simulink model "CiMappedEngine"  (R2021b)
settings: Solver=VariableStepAuto  StartTime=0.0  StopTime=inf  RelTol=1e-3  EnableMultiTasking=on
model workspace (MAT data in the model file):
  AccPwrbp = Simulink.Parameter
  AccPwrbp.Value = [0 0]
  AccPwrbp.DataType = 'double'
  AccPwrbp.Complexity = 'real'
  AccPwrbp.Dimensions = [1 2]
  AccSpdbp = Simulink.Parameter
  AccSpdbp.Value = [300 750]
  AccSpdbp.DataType = 'double'
  AccSpdbp.Complexity = 'real'
  AccSpdbp.Dimensions = [1 2]
  Cps = Simulink.Parameter
  Cps.Value = 2
  Cps.DataType = 'double'
  Cps.Complexity = 'real'
  Cps.Dimensions = [1 1]
  NCyl = Simulink.Parameter
  NCyl.Value = 4
  NCyl.DataType = 'double'
  NCyl.Complexity = 'real'
  NCyl.Dimensions = [1 1]
  Pstd = Simulink.Parameter
  Pstd.Value = 101325
  Pstd.DataType = 'double'
  Pstd.Complexity = 'real'
  Pstd.Dimensions = [1 1]
  Rair = Simulink.Parameter
  Rair.Value = 287.05
  Rair.DataType = 'double'
  Rair.Complexity = 'real'
  Rair.Dimensions = [1 1]
  Sinj = Simulink.Parameter
  Sinj.Value = 6.45161290323
  Sinj.DataType = 'double'
  Sinj.Complexity = 'real'
  Sinj.Dimensions = [1 1]
  TimeCnstECP = Simulink.Parameter
  TimeCnstECP.Value = 0.125
  TimeCnstECP.DataType = 'double'
  TimeCnstECP.Complexity = 'real'
  TimeCnstECP.Dimensions = [1 1]
  TimeCnstEGR = Simulink.Parameter
  TimeCnstEGR.Value = 0.125
  TimeCnstEGR.DataType = 'double'
  TimeCnstEGR.Complexity = 'real'
  TimeCnstEGR.Dimensions = [1 1]
  TimeCnstETC = Simulink.Parameter
  TimeCnstETC.Value = 0.085
  TimeCnstETC.DataType = 'double'
  TimeCnstETC.Complexity = 'real'
  TimeCnstETC.Dimensions = [1 1]
  TimeCnstICP = Simulink.Parameter
  TimeCnstICP.Value = 0.125
  TimeCnstICP.DataType = 'double'
  TimeCnstICP.Complexity = 'real'
  TimeCnstICP.Dimensions = [1 1]
  TimeCnstIVL = Simulink.Parameter
  TimeCnstIVL.Value = 0.125
  TimeCnstIVL.DataType = 'double'
  TimeCnstIVL.Complexity = 'real'
  TimeCnstIVL.Dimensions = [1 1]
  TimeCnstSWVA = Simulink.Parameter
  TimeCnstSWVA.Value = 0.125
  TimeCnstSWVA.DataType = 'double'
  TimeCnstSWVA.Complexity = 'real'
  TimeCnstSWVA.Dimensions = [1 1]
  TimeCnstVCR = Simulink.Parameter
  TimeCnstVCR.Value = 0.125
  TimeCnstVCR.DataType = 'double'
  TimeCnstVCR.Complexity = 'real'
  TimeCnstVCR.Dimensions = [1 1]
  TimeCnstVGT = Simulink.Parameter
  TimeCnstVGT.Value = 0.15
  TimeCnstVGT.DataType = 'double'
  TimeCnstVGT.Complexity = 'real'
  TimeCnstVGT.Dimensions = [1 1]
  TimeCnstVIRL = Simulink.Parameter
  TimeCnstVIRL.Value = 0.125
  TimeCnstVIRL.DataType = 'double'
  TimeCnstVIRL.Complexity = 'real'
  TimeCnstVIRL.Dimensions = [1 1]
  TimeCnstWGA = Simulink.Parameter
  TimeCnstWGA.Value = 0.15
  TimeCnstWGA.DataType = 'double'
  TimeCnstWGA.Complexity = 'real'
  TimeCnstWGA.Dimensions = [1 1]
  Tstd = Simulink.Parameter
  Tstd.Value = 293.15
  Tstd.DataType = 'double'
  Tstd.Complexity = 'real'
  Tstd.Dimensions = [1 1]
  Vd = Simulink.Parameter
  Vd.Value = 0.0015
  Vd.DataType = 'double'
  Vd.Complexity = 'real'
  Vd.Dimensions = [1 1]
  f_air = Simulink.Parameter
  f_air.Value = [0 0 0 0 0 0 0 0 0 0 0 0 ... (320 elements, 20x16)]
  f_air.DataType = 'double'
  f_air.Complexity = 'real'
  f_air.Dimensions = [20 16]
  f_air_3d = Simulink.Parameter
  f_air_3d.Value = [0 0 0 0 0 0 0 0 0 0 0 0 ... (960 elements, 20x16x3)]
  f_air_3d.DataType = 'double'
  f_air_3d.Complexity = 'real'
  f_air_3d.Dimensions = [20 16 3]
  f_co = Simulink.Parameter
  f_co.Value = [0 0 0 0 0 0 0 0 0 0 0 0 ... (320 elements, 20x16)]
  f_co.DataType = 'double'
  f_co.Complexity = 'real'
  f_co.Dimensions = [20 16]
  f_co2 = Simulink.Parameter
  f_co2.Value = [0 0 0 0 0 0 0 0 0 0 0 0 ... (320 elements, 20x16)]
  f_co2.DataType = 'double'
  f_co2.Complexity = 'real'
  f_co2.Dimensions = [20 16]
  f_co2_3d = Simulink.Parameter
  f_co2_3d.Value = [0 0 0 0 0 0 0 0 0 0 0 0 ... (960 elements, 20x16x3)]
  f_co2_3d.DataType = 'double'
  f_co2_3d.Complexity = 'real'
  f_co2_3d.Dimensions = [20 16 3]
  f_co_3d = Simulink.Parameter
  f_co_3d.Value = [0 0 0 0 0 0 0 0 0 0 0 0 ... (960 elements, 20x16x3)]
  f_co_3d.DataType = 'double'
  f_co_3d.Complexity = 'real'
  f_co_3d.Dimensions = [20 16 3]
  f_eff = Simulink.Parameter
  f_eff.Value = [0 0 0 0 0 0 0 0 0 0 0 0 ... (320 elements, 20x16)]
  f_eff.DataType = 'double'
  f_eff.Complexity = 'real'
  f_eff.Dimensions = [20 16]
  f_eff_3d = Simulink.Parameter
  f_eff_3d.Value = [0 0 0 0 0 0 0 0 0 0 0 0 ... (960 elements, 20x16x3)]
  f_eff_3d.DataType = 'double'
  f_eff_3d.Complexity = 'real'
  f_eff_3d.Dimensions = [20 16 3]
  f_fuel = Simulink.Parameter
  f_fuel.Value = [0 0 0 0 0 0 0 0 0 0 0 0 ... (320 elements, 20x16)]
  f_fuel.DataType = 'double'
  f_fuel.Complexity = 'real'
  f_fuel.Dimensions = [20 16]
  f_fuel_3d = Simulink.Parameter
  f_fuel_3d.Value = [0 0 0 0 0 0 0 0 0 0 0 0 ... (960 elements, 20x16x3)]
  f_fuel_3d.DataType = 'double'
  f_fuel_3d.Complexity = 'real'
  f_fuel_3d.Dimensions = [20 16 3]
  f_hc = Simulink.Parameter
  f_hc.Value = [0 0 0 0 0 0 0 0 0 0 0 0 ... (320 elements, 20x16)]
  f_hc.DataType = 'double'
  f_hc.Complexity = 'real'
  f_hc.Dimensions = [20 16]
  f_hc_3d = Simulink.Parameter
  f_hc_3d.Value = [0 0 0 0 0 0 0 0 0 0 0 0 ... (960 elements, 20x16x3)]
  f_hc_3d.DataType = 'double'
  f_hc_3d.Complexity = 'real'
  f_hc_3d.Dimensions = [20 16 3]
  f_nox = Simulink.Parameter
  f_nox.Value = [0 0 0 0 0 0 0 0 0 0 0 0 ... (320 elements, 20x16)]
  f_nox.DataType = 'double'
  f_nox.Complexity = 'real'
  f_nox.Dimensions = [20 16]
  f_nox_3d = Simulink.Parameter
  f_nox_3d.Value = [0 0 0 0 0 0 0 0 0 0 0 0 ... (960 elements, 20x16x3)]
  f_nox_3d.DataType = 'double'
  f_nox_3d.Complexity = 'real'
  f_nox_3d.Dimensions = [20 16 3]
  f_pm = Simulink.Parameter
  f_pm.Value = [0  0  0  0  0  0  0  0  0  0  0  0  0  0  0  0; 0  0  0  0  0  0  0  0  0  0  0  0  0  0  0  0; 0  0  0  0  0  0  0  0  0  0  0  0  0  0  0  0; 0  0  0  0  0  0  0  0  0  0  0  0  0  0  0  0; 0  0  0  0  0  0  0  0  0  0  0  0  0  0  0  0; 0  0  0  0  0  0  0  0  0  0  0  0  0  0  0  0; 0  0  0  0  0  0  0  0  0  0  0  0  0  0  0  0; 0  0  0  0  0  0  0  0  0  0  0  0  0  0  0  0; 0  0  0  0  0  0  0  0  0  0  0  0  0  0  0  0; 0  0  0  0  0  0  0  0  0  0  0  0  0  0  0  0; 0  0  0  0  0  0  0  0  0  0  0  0  0  0  0  0; 0  0  0  0  0  0  0  0  0  0  0  0  0  0  0  0; 0  0  0  0  0  0  0  0  0  0  0  0  0  0  0  0; 0  0  0  0  0  0  0  0  0  0  0  0  0  0  0  0; 0  0  0  0  0  0  0  0  0  0  0  0  0  0  0  0; 0  0  0  0  0  0  0  0  0  0  0  0  0  0  0  0; 0  0  0  0  0  0  0  0  0  0  0  0  0  0  0  0; 0  0  0  0  0  0  0  0  0  0  0  0  0  0  0  0; 0  0  0  0  0  0  0  0  0  0  0  0  0  0  0  0; 0  0  0  0  0  0  0  0  0  0  0  0  0  0  0  0]
  f_pm.DataType = 'double'
  f_pm.Complexity = 'real'
  f_pm.Dimensions = [20 16]
  f_pm_3d = Simulink.Parameter
  f_pm_3d.Value = reshape([0 0 0 0 0 0 0 0 0 0 0 0 0 0 0 0 0 0 0 0 0 0 0 0 0 0 0 0 0 0 0 0 0 0 0 0 0 0 0 0 0 0 0 0 0 0 0 0 0 0 0 0 0 0 0 0 0 0 0 0 0 0 0 0 0 0 0 0 0 0 0 0 0 0 0 0 0 0 0 0 0 0 0 0 0 0 0 0 0 0 0 0 0 0 0 0 0 0 0 0 0 0 0 0 0 0 0 0 0 0 0 0 0 0 0 0 0 0 0 0 0 0 0 0 0 0 0 0 0 0 0 0 0 0 0 0 0 0 0 0 0 0 0 0 0 0 0 0 0 0 0 0 0 0 0 0 0 0 0 0 0 0 0 0 0 0 0 0 0 0 0 0 0 0 0 0 0 0 0 0 0 0 0 0 0 0 0 0 0 0 0 0 0 0 0 0 0 0 0 0 0 0 0 0 0 0 0 0 0 0 0 0 0 0 0 0 0 0 0 0 0 0 0 0 0 0 0 0 0 0 0 0 0 0 0 0 0 0 0 0 0 0 0 0 0 0 0 0 0 0 0 0 0 0 0 0 0 0 0 0 0 0 0 0 0 0 0 0 0 0 0 0 0 0 0 0 0 0 0 0 0 0 0 0 0 0 0 0 0 0 0 0 0 0 0 0 0 0 0 0 0 0 0 0 0 0 0 0 0 0 0 0 0 0 0 0 0 0 0 0 0 0 0 0 0 0 0 0 0 0 0 0 0 0 0 0 0 0 0 0 0 0 0 0 0 0 0 0 0 0 0 0 0 0 0 0 0 0 0 0 0 0 0 0 0 0 0 0 0 0 0 0 0 0 0 0 0 0 0 0 0 0 0 0 0 0 0 0 0 0 0 0 0 0 0 0 0 0 0 0 0 0 0 0 0 0 0 0 0 0 0 0 0 0 0 0 0 0 0 0 0 0 0 0 0 0 0 0 0 0 0 0 0 0 0 0 0 0 0 0 0 0 0 0 0 0 0 0 0 0 0 0 0 0 0 0 0 0 0 0 0 0 0 0 0 0 0 0 0 0 0 0 0 0 0 0 0 0 0 0 0 0 0 0 0 0 0 0 0 0 0 0 0 0 0 0 0 0 0 0 0 0 0 0 0 0 0 0 0 0 0 0 0 0 0 0 0 0 0 0 0 0 0 0 0 0 0 0 0 0 0 0 0 0 0 0 0 0 0 0 0 0 0 0 0 0 0 0 0 0 0 0 0 0 0 0 0 0 0 0 0 0 0 0 0 0 0 0 0 0 0 0 0 0 0 0 0 0 0 0 0 0 0 0 0 0 0 0 0 0 0 0 0 0 0 0 0 0 0 0 0 0 0 0 0 0 0 0 0 0 0 0 0 0 0 0 0 0 0 0 0 0 0 0 0 0 0 0 0 0 0 0 0 0 0 0 0 0 0 0 0 0 0 0 0 0 0 0 0 0 0 0 0 0 0 0 0 0 0 0 0 0 0 0 0 0 0 0 0 0 0 0 0 0 0 0 0 0 0 0 0 0 0 0 0 0 0 0 0 0 0 0 0 0 0 0 0 0 0 0 0 0 0 0 0 0 0 0 0 0 0 0 0 0 0 0 0 0 0 0 0 0 0 0 0 0 0 0 0 0 0 0 0 0 0 0 0 0 0 0 0 0 0 0 0 0 0 0 0 0 0 0 0 0 0 0 0 0 0 0 0 0 0 0 0 0 0 0 0 0 0 0 0 0 0 0 0 0 0 0 0 0 0 0 0 0 0 0 0 0 0 0 0 0 0 0 0 0 0 0 0 0 0 0 0 0 0 0 0 0 0 0 0 0 0 0 0 0 0 0 0 0 0 0 0 0 0 0 0 0 0 0 0 0 0 0 0 0 0 0 0 0 0 0 0 0 0 0 0 0 0 0 0 0 0 0 0 0 0 0 0 0 0 0 0 0 0 0 0 0 0 0 0 0 0 0 0 0 0 0 0 0 0 0 0 0 0 0 0 0 0 0 0 0 0 0 0 0 0 0 0 0 0 0 0 0 0 0 0 0 0 0 0 0 0 0 0 0 0 0 0 0 0 0 0 0 0 0 0 0 0 0 0 0 0 0 0 0 0 0 0 0 0 0 0 0 0 0 0 0 0 0 0 0 0 0 0 0 0 0], [20 16 3])
  f_pm_3d.DataType = 'double'
  f_pm_3d.Complexity = 'real'
  f_pm_3d.Dimensions = [20 16 3]
  f_tbrake = Simulink.Parameter
  f_tbrake.Value = [0 15 15 15 15 15 15 15 15 15 15 15 ... (320 elements, 20x16)]
  f_tbrake.DataType = 'double'
  f_tbrake.Complexity = 'real'
  f_tbrake.Dimensions = [20 16]
  f_tbrake_3d = Simulink.Parameter
  f_tbrake_3d.Value = [0 4.32139921766 20.7572447114 35.9627269415 49.855265726 62.5657141177 74.4770044016 86.1003984024 97.7334079818 109.479762957 121.326441846 133.101497884 ... (960 elements, 20x16x3)]
  f_tbrake_3d.DataType = 'double'
  f_tbrake_3d.Complexity = 'real'
  f_tbrake_3d.Dimensions = [20 16 3]
  f_tbrake_f_bpt = Simulink.Parameter
  f_tbrake_f_bpt.Value = [0 2.63157894737 5.26315789474 7.89473684211 10.5263157895 13.1578947368 15.7894736842 18.4210526316 21.0526315789 23.6842105263 26.3157894737 28.9473684211 31.5789473684 34.2105263158 36.8421052632 39.4736842105 42.1052631579 44.7368421053 47.3684210526 50]
  f_tbrake_f_bpt.DataType = 'double'
  f_tbrake_f_bpt.Complexity = 'real'
  f_tbrake_f_bpt.Dimensions = [1 20]
  f_tbrake_n_bpt = Simulink.Parameter
  f_tbrake_n_bpt.Value = [0 1000 1285.71428571 1571.42857143 1857.14285714 2142.85714286 2428.57142857 2714.28571429 3000 3285.71428571 3571.42857143 3857.14285714 4142.85714286 4428.57142857 4714.28571429 5000]
  f_tbrake_n_bpt.DataType = 'double'
  f_tbrake_n_bpt.Complexity = 'real'
  f_tbrake_n_bpt.Dimensions = [1 16]
  f_tbrake_t_bpt = Simulink.Parameter
  f_tbrake_t_bpt.Value = [0 4.017 21.26 37.37 52.22 65.88 78.77 91.44 104.2 116.8 129.3 141.4 153.4 165.7 178.4 191.7 205.6 219.7 233.5 246.7]
  f_tbrake_t_bpt.DataType = 'double'
  f_tbrake_t_bpt.Complexity = 'real'
  f_tbrake_t_bpt.Dimensions = [1 20]
  f_texh = Simulink.Parameter
  f_texh.Value = [530.615953519 585.141308787 621.791548793 637.74644696 668.027558986 729.99378178 762.870339995 814.420601609 844.420048857 859.04703204 894.926983859 943.665474082 ... (320 elements, 20x16)]
  f_texh.DataType = 'double'
  f_texh.Complexity = 'real'
  f_texh.Dimensions = [20 16]
  f_texh_3d = Simulink.Parameter
  f_texh_3d.Value = [358.711368346 410.521929896 465.556483184 518.480956339 566.158596806 618.256764358 675.886138918 720.044246232 742.940029896 751.128194054 760.390444558 779.777710435 ... (960 elements, 20x16x3)]
  f_texh_3d.DataType = 'double'
  f_texh_3d.Complexity = 'real'
  f_texh_3d.Dimensions = [20 16 3]
libraries: autolibpowerinfoutils x1, autolibsharedmappedengines x1
(part 1 of 2)
settings Model: DataDictionary=CiMappedEngine.sldd  ModifiedByFormat=The MathWorks, Inc.  Creator=The MathWorks, Inc.  LastModifiedBy=The MathWorks, Inc.
settings SolverCC: AlgebraicLoopSolver=TrustRegion  DecoupledContinuousIntegration=on
settings DataIOCC: DSMLogging=off  ReturnWorkspaceOutputs=off
settings DebuggingCC: SFMachineParentedDataDiag=warning  ArithmeticOperatorsInVariantConditions=warning
settings SFSimCC: SimUseLocalCustomCode=off  CustomCodeUndefinedFunction=UseInterfaceOnly
settings RTWCC: RTWUseLocalCustomCode=off
settings CodeAppCC: StateflowObjectComments=on
settings GRTTargetCC: TargetLangStandard=C89/C90 (ANSI)
settings ConfigComp: CovMetricSettings=dsw  CovSaveCumulativeToWorkspaceVar=on  CovSaveSingleToWorkspaceVar=on  CovExternalEMLEnable=off
settings SimscapeCC: SimscapeNormalizeSystem=off  SimscapeNominalValues={1, 'bar'; 1, 'cm^3/s'; 1, 'bar*kg/s'; 1, 'kJ/kg'; 1, 'kW'}

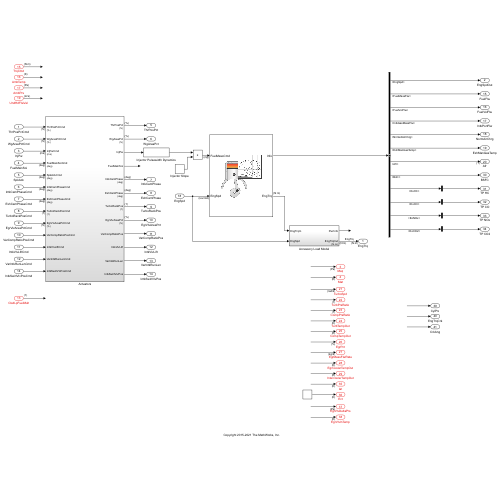
[thumbnail: Simulink's stored preview of the top-level diagram]
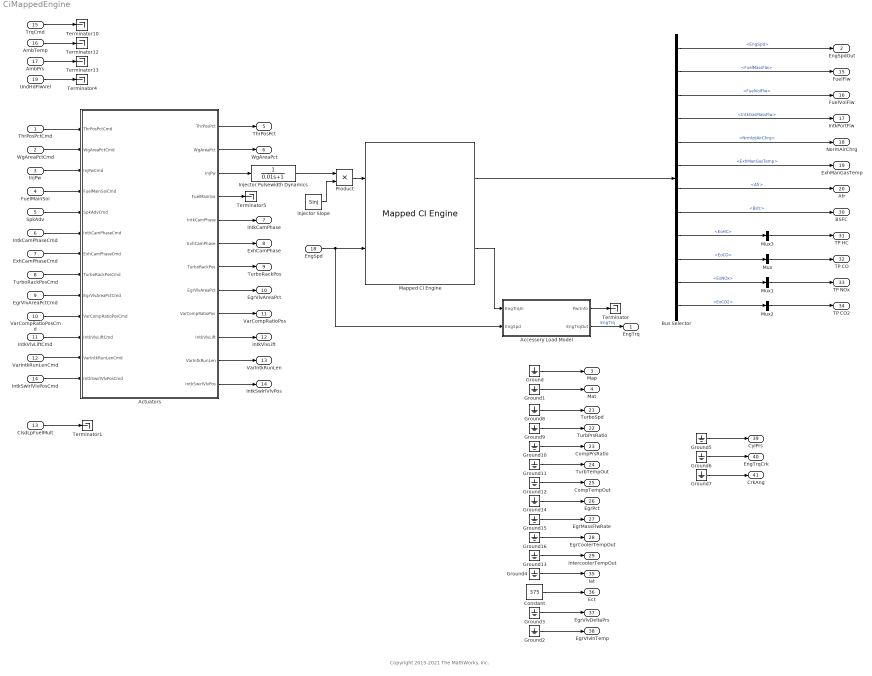
== system CiMappedEngine ==
  note: Copyright 2015-2021 The MathWorks, Inc.
  ThrPosPctCmd : Inport
  WgAreaPctCmd : Inport  Port=2
  InjPw : Inport  Port=3
  FuelMainSoi : Inport  Port=4
  SpkAdv : Inport  Port=5
  IntkCamPhaseCmd : Inport  Port=6
  ExhCamPhaseCmd : Inport  Port=7
  TurboRackPosCmd : Inport  Port=8
  EgrVlvAreaPctCmd : Inport  Port=9
  VarCompRatioPosCmd : Inport  Port=10
  IntkVlvLiftCmd : Inport  Port=11
  VarIntkRunLenCmd : Inport  Port=12
  ClsdLpFuelMult : Inport  Port=13  Unit=1
  IntkSwirlVlvPosCmd : Inport  Port=14
  TrqCmd : Inport  Port=15  Unit=N*m
  AmbTemp : Inport  Port=16  Unit=K
  AmbPrs : Inport  Port=17  Unit=Pa
  EngSpd : Inport  Port=18  Interpolate=off
  UndHdFlwVel : Inport  Port=19  Unit=m/s
  Accessory Load Model : Subsystem
  Actuators : Subsystem
  Bus Selector : BusSelector  OutputSignals=EngSpd,FuelMassFlw,FuelVolFlw,IntkGasMassFlw,NrmlzdAirChrg,ExhManGasTemp,Afr,Bsfc,EoHC,EoCO,EoNOx,EoCO2
  Constant : Constant  Value=375
  Ground{,1..16} (17 alike) : Ground
  Injector Pulsewidth Dynamics : TransferFcn  Denominator=[0.01 1]
  Injector Slope : Constant  Value=Sinj
  Mapped CI Engine : autolibsharedmappedengines/Mapped CI Engine  InputCmdPopup=Fuel mass  TurboLagCheckbox=off  EngTmpInpEnbl=off  rowVarName=TrqCmd  f_tbrake_f_bpt=f_tbrake_f_bpt  f_tbrake_t_bpt=f_tbrake_t_bpt  colVarName=EngSpd  f_tbrake_n_bpt=f_tbrake_n_bpt  f_tbrake_engtmp_bpt=[0 1000 1285.71428571429 1571.42857142857 1857.14285714286 2142.85714285714 2428.57142857143 2714.28571428571 3000 3285.71428571429 3571.42857142857 3857.14285714286 4142.85714285714 4428.57142857143 4714.28571428571 5000]  NCyl=NCyl  Cps=Cps  Vd=Vd  Lhv=45e6  Sg=0.832  Rair=Rair  Pstd=Pstd  Tstd=Tstd  Use1=on  Use2=on  Use3=on  Use4=on  Use5=on  Use6=on  Use7=on  Use8=on  Use9=on  Use10=off  f_tbrake_bst=[90, 95, 95, 95, 96, 100, 104, 104, 104, 100, 95, 85, 75, 67, 60, 55]  tau_nat=0.1  tau_bst_rising=1.0  tau_bst_falling=0.7  f_blend_frac=0.01  Name1=Brake Torque  f_tbrake=f_tbrake  f_tbrake_3d=cat(3,[0 -13.1081458684774 -14.1037949635308 -15.5978222223895 -17.1468243988479 -18.57688227287 -19.9284644067992 -21.2542794863055 -22.5937120686825 -24.0017516696912 -25.5203729932636 -27.1667334739623 -28.9776139270543 -31.0652059053262 -33.6382508909905 -36.9873078874202;4.32139921766168 4.32139921766168 4.01696946242645 3.01657627710533 1.85358637804622 0.731516929734549 -0.4275387192502 -1.6561494194378 -2.95770994431816 -4.36637302182332 -5.88102944693574 -7.45086843033805 -9.05557392067087 -10.7763270640777 -12.796196773429 -15.3493054793365;20.757244711379 20.757244711379 21.2571513067777 20.7978892952266 19.9910981679013 19.1178286650763 18.1132099278104 16.9543909701551 15.6490277189844 14.1813864135569 12.6063311068736 11.047099076305 9.56356301296286 8.06856710184566 6.37897429143581 4.32789906798446;35.9627269414642 35.9627269414642 37.3688456485072 37.4967194297404 37.0204872778024 36.3613948045835 35.5253088841127 34.4682997931625 33.1775441596392 31.6622717238732 30.0361023542073 28.4879672009938 27.0975462675126 25.7330173462773 24.1825303780978 22.3468615101609;49.8552657259726 49.8552657259726 52.2167310328196 52.9733200758864 52.8662249930047 52.4835369255407 51.8917326649162 51.0033454025654 49.7832430749781 48.2789577545489 46.6575307752233 45.1520123081703 43.8459468590103 42.5572123684317 41.0363966513775 39.2223005091444;62.5657141177372 62.5657141177372 65.8831947231727 67.3435083597075 67.7482462698726 67.8043747818398 67.5850553575219 66.9435552010083 65.8425982505031 64.3910827013451 62.8078461464009 61.3518293888112 60.1077185922706 58.8589256293869 57.319516534669 55.4366133009561;74.477004401576 74.477004401576 78.7701323679482 81.0576508161983 82.1550115553721 82.8010970398817 83.0434289470775 82.6817940293035 81.6963304630852 80.2758690996741 78.6966647443712 77.2463474522679 76.0244210658268 74.7962055302467 73.2304818257695 71.2491878151604;86.1003984024147 86.1003984024147 91.4403848598737 94.6662578802864 96.5423763308834 97.7951601239239 98.4662457785871 98.3255389688887 97.3704373723042 95.8764879743608 94.2178248871414 92.7449049403045 91.560940932338 90.3786230785299 88.8022437200717 86.7312355288638;97.7334079817966 97.7334079817966 104.159640567149 108.333038149937 110.951645304697 112.751774515793 113.767119577956 113.736058315812 112.652011363998 110.885495354204 109.00563172831 107.50897096566 106.468900898909 105.447451722756 103.936744797267 101.836124688201;109.479762957418 109.479762957418 116.819239580331 121.785496063185 125.100419113855 127.517149489911 128.937109713723 128.978763347179 127.598490805448 125.286894087135 122.924794214455 121.283173749861 120.428652893331 119.688104302635 118.358109739931 116.328046918923;121.326441846396 121.326441846396 129.256746784122 134.801128987357 138.834183316905 142.084246404129 144.125534715133 144.323033261273 142.583968288345 139.561104144292 136.474675856478 134.450177681175 133.638504705164 133.121882385945 131.951673587603 130.013338129768;133.101497884419 133.101497884419 141.390423214992 147.492975799703 152.341446310031 156.513845250296 159.270404298858 159.701130755565 157.676228517122 154.055833011852 150.345084498928 147.936876100182 147.055031208233 146.57504282138 145.352051741223 143.327096283665;144.820899208063 144.820899208063 153.421621226276 160.170390947986 165.811081311634 170.679187177046 174.011429217703 174.723297653528 172.66129491056 168.876865408438 165.011029375467 162.478515988541 161.481832233675 160.830603115659 159.333139273686 157.000941329443;156.736480114968 156.736480114968 165.665608236336 172.981857305465 179.187187414613 184.464635460139 188.162745737646 189.162853683952 187.38585429464 184.016652748413 180.526272843455 178.002164899037 176.608934842436 175.45436155568 173.584473896243 170.951232344112;169.114710642361 169.114710642361 178.391434699741 186.176266646156 192.786027371817 198.285653474534 202.073246296265 203.186779695165 201.750788334907 198.96643821215 195.929170221711 ...(+12274 chars)])  Name2=Air Mass Flow  f_air=f_air  f_air_3d=cat(3,[0 0.00309706924950592 0.00452015548895638 0.00626693492213078 0.00879912183278348 0.0118780141352622 0.0146086872326241 0.0164283363560914 0.017430833463342 0.0179780359688698 0.0183296451622608 0.0185647242912905 0.0186520238218037 0.0185206414129648 0.0181086367688216 0.0174012027671944;0 0.00602292528585861 0.00770048695740641 0.00909327842187188 0.0120300250825315 0.0165547686351833 0.0195929621698111 0.0205166972641812 0.0205599898366506 0.0207203034276991 0.0211816497894974 0.0218000682616549 0.0224177900393616 0.0228313059997907 0.022838545013414 0.0223621006077339;0 0.00872840998619654 0.0119344185519278 0.0150347158665953 0.0186401194316719 0.0220516764842476 0.0232455963198542 0.0227496747610248 0.022315206695101 0.0227059865534211 0.0235552063657731 0.0247029468037314 0.0262251280736842 0.0276235809443034 0.0283154367096376 0.0283212514239343;0 0.0104882072017092 0.0149369369892934 0.0194071452576307 0.0234570953719028 0.0264743743207795 0.0278624533425652 0.0279142745177744 0.0275369343940129 0.0274156787405589 0.0276419826170279 0.028751250915015 0.0310753059304267 0.0334431313520856 0.0347160350646922 0.0352041887413915;0 0.011712168284924 0.0163701147244402 0.0205936040826631 0.024568631705785 0.0286183696627147 0.0321435952324048 0.034217055691985 0.0347312239715439 0.034496131683675 0.0346154869246281 0.0357155943731093 0.0376532165828575 0.0397890303933338 0.041465041333155 0.0422265141888633;0 0.0118312143050573 0.0161536266038965 0.0199257826871529 0.0236447392965077 0.0278874214850712 0.0320911410431683 0.0355319414463786 0.0381473109012507 0.0402474553755304 0.0418777340103424 0.0430635720676062 0.044104298120767 0.0452740851072815 0.0464766914282441 0.0473016169107081;0 0.0110465687603505 0.0147448001879976 0.0186982152653005 0.0233180272070577 0.02848967544271 0.0332213005321568 0.0370211588830352 0.0405545130029438 0.044572205134237 0.0483929460850711 0.0506432109795243 0.0511287512595987 0.0512056237163403 0.0520782826150034 0.0532844037021472;0 0.0104431005689455 0.0140412319781156 0.0186656040327574 0.0243808115038222 0.0304790901592309 0.0358563735218778 0.0398156150298808 0.0431173259508535 0.0469471574428406 0.0509987494297762 0.0536398238059855 0.0543064471273892 0.0546047048338575 0.056061016585052 0.0580171322968633;0 0.0108025838625983 0.0147329075783379 0.0199272160885801 0.0269494950175881 0.0350856622579705 0.0423805976180197 0.0475930434283361 0.0511546617444798 0.0538624225439131 0.0553835460317609 0.0555838102527836 0.0555667873119217 0.056594819532664 0.0588984420072796 0.0617150043278395;0 0.01183615404291 0.015579473332316 0.0207476894033608 0.0291566563357895 0.0404435443970542 0.0507984356999528 0.0587530704305265 0.0649619731202889 0.0698463364144272 0.0724789010286908 0.0725501004086276 0.0711596039900798 0.0695425955723599 0.0686753046594181 0.0693454311429488;0 0.0127240149300819 0.0166943434305672 0.0213167267720966 0.0289502837647639 0.0400653409995224 0.0513974226551378 0.0604623088982535 0.0678845803192903 0.0753268542302593 0.0820105776211095 0.0855945811173189 0.0853773765956796 0.0831281579249428 0.081073849758615 0.080081315740193;0 0.0110641453709759 0.0153408643765708 0.0205300836592455 0.0288449359807962 0.0405948104237211 0.0521701453289181 0.0615930540891253 0.0695902332854493 0.0773195773497623 0.0841151408595659 0.088334695168896 0.089836067046592 0.0903700280065862 0.0909243501674699 0.0904976630313823;0 0.00833019140075226 0.0135692203293849 0.0205158026876127 0.029849570119091 0.040810538170541 0.0510111942628966 0.0598705369646537 0.0681187978770399 0.0760999983843794 0.0825339047146241 0.0867122889636778 0.0895837553206919 0.0920372076390418 0.0940819738186311 0.0954699432157815;0 0.00655239324915465 0.0124582375744647 0.019731165806625 0.0283852357889038 0.038223674378621 0.049417712197541 0.0598093990036953 0.0683274458944638 0.075112746920361 0.0800000023035051 0.0829602155432646 0.0850309276879992 0.0876816601880811 0.0912763887167288 ...(+13141 chars)])  Name3=Fuel Flow  f_fuel=f_fuel  f_fuel_3d=cat(3,[0 0 0 0 0 0 1.96872590895162e-08 1.11497559089192e-07 2.08845127798106e-07 2.82196894845497e-07 3.36789183807035e-07 3.85963069087249e-07 4.43703799512474e-07 5.16303552365966e-07 6.18958920559444e-07 7.66022406381668e-07;0 8.65785362426501e-05 0.00011203764940267 0.000137411179243721 0.00016270746005005 0.000187945932561446 0.00021312794139946 0.0002382669520308 0.000263366151267778 0.000288441610892002 0.000313504671335018 0.000338563835699193 0.000363629535167578 0.000388708193714062 0.000413810734167462 0.000438953321603612;0 0.000174726035507858 0.000225152899075032 0.000275508155686899 0.000325799742757026 0.000376033006192685 0.000426224614562359 0.000476378444759466 0.00052650775641107 0.00057661136482858 0.000626701339027024 0.000676788018376088 0.000726877918663027 0.000776982406974879 0.000827105108458734 0.000877258289084099;0 0.000262751467992024 0.00033815711141714 0.000413509147749243 0.000488810553518419 0.000564063749931979 0.00063928056610551 0.000714470811260552 0.000789634562401864 0.000864779715478911 0.00093991739471757 0.00101505165767627 0.00109018850480272 0.00116533546923552 0.00124049316997444 0.00131567174054954;0 0.000350674622437212 0.000451079528986024 0.000551436546045139 0.000651750832933373 0.000752042172469353 0.000852303056689121 0.00095253536480496 0.00105275214616171 0.00115295860006142 0.0012531576082591 0.00135334897972371 0.00145354034681151 0.00155374157057415 0.00165395024017036 0.00175417640620197;0 0.000438523155398598 0.000563925299253614 0.00068929628290271 0.000814645829677503 0.000939976999036283 0.001065288419702 0.00119058587147412 0.0013158694017402 0.00144114084528669 0.00156640851566576 0.0016916722751574 0.00181693265390974 0.00194219580045656 0.00206746569238982 0.00219275425952363;0 0.000526315425106774 0.000676728986990437 0.000827125576794928 0.000977509956968386 0.00112788874103488 0.00127826025858348 0.00142862216689251 0.00157897837839604 0.00172932766397965 0.00187967288170457 0.00203001238929626 0.00218034633484077 0.00233068458827493 0.00248102887035893 0.00263137738480869;0 0.000614090293790132 0.000789508746068303 0.000964932673154394 0.00114036147974239 0.00131579049815924 0.00149122146693545 0.00166665161834229 0.0018420830255848 0.00201751320081695 0.00219293915270003 0.00236836178159738 0.00254378375898177 0.00271920464503755 0.00289462481590337 0.00307005046750055;0 0.000701854437168888 0.000902286333293199 0.00110273789235218 0.00130320355815633 0.00150368554903504 0.00170418578418384 0.00190468941205035 0.00210519697462961 0.00230570553537478 0.0025062157636349 0.00270672441780583 0.00290722747290807 0.00310772903092585 0.00330823075338495 0.00350873484232527;0 0.000789649340075805 0.0010150845509588 0.00124055848345417 0.00146606558137245 0.00169159899277097 0.00191715641046872 0.00214272626450072 0.00236830926864185 0.00259390116245577 0.00281949040707559 0.00304508145248784 0.00327067513685969 0.00349626254985207 0.00372184957344385 0.0039474323233373;0 0.000877488592369892 0.00112793274528237 0.00137842091388439 0.00162895825749475 0.00187953790343879 0.00213014403908549 0.0023807781378913 0.00263143096817038 0.00288209397350937 0.0031327661795019 0.00338344231576459 0.00363411526528075 0.00388478536124402 0.00413545265696539 0.00438611177099695;0 0.000965411294698122 0.00124084233073851 0.00151633453527839 0.0017918942582486 0.00206750600688409 0.00234316285075658 0.00261885261867168 0.00289456620925925 0.00317029654400497 0.00344604094255091 0.00372179266401898 0.00399754312534031 0.00427329087379054 0.00454903339486812 0.00482476409430018;0 0.0010534117250146 0.00135382536745709 0.00165432071941838 0.00195489381219168 0.0022555293855071 0.00255621411457967 0.00285694714347189 0.00315771657791031 0.00345850732940484 0.00375931514196172 0.00406013514206826 0.00436095638616358 0.0046617732232831 0.00496258457239849 0.00526338302180174;0 0.00114152016247886 0.00146691663641427 0.00179239333752689 0.00211796534690249 0.00244360868792483 ...(+13971 chars)])  Name4=Exhaust Temperature  f_texh=f_texh  f_texh_3d=cat(3,[358.711368346279 358.711368346279 367.983969839492 375.766236578521 379.824873013623 380.377581918888 381.168020674094 384.445628826361 389.975238414473 397.276334747317 406.687273458426 418.723655106797 433.343123892387 449.95713948592 467.887943023565 486.766068837338;410.521929895625 410.521929895625 418.333326741241 425.972726120476 430.142630320378 430.676036782825 433.565609920626 439.830692307499 446.677697654088 452.935492545412 459.921840004908 469.184147095924 481.106853505583 495.16688690855 510.625205052308 527.104289154894;465.556483183975 465.556483183975 470.789185946812 475.838502443986 480.295227783728 485.406910889802 495.495051944124 508.573634165955 519.57749983902 526.850757499387 532.455117721457 538.704931547602 546.67711884581 556.710936307477 568.417449771026 581.104011694485;518.480956338607 518.480956338607 520.899294741741 523.582135138291 528.595311716542 536.846832033099 550.734399138879 568.993556445828 586.848331191129 600.477075260956 609.4895047716 615.505834518885 620.86855927714 627.910927144035 637.072100901679 647.109616946413;566.158596806175 566.158596806175 567.687323012922 572.746317112909 580.726768000975 588.013457446177 597.926992283215 614.220587792806 634.624060621759 653.584855786604 667.720901691748 677.333709356163 684.916260551597 693.10564253556 702.779084224323 713.371213106786;618.256764358386 618.256764358386 624.477092679185 633.413924976204 641.337589870685 643.8930379857 648.163836293112 659.880379116932 675.9331795421 690.676983743342 703.48679807145 716.671213932218 730.807374933275 744.672663864793 757.311023892644 769.273185572513;675.886138917862 675.886138917862 690.728265001459 698.761147883829 697.795213788686 691.167357063837 691.393891761148 702.947342129308 717.508872010719 726.807220251821 733.985585412432 746.79008634134 766.115681043826 785.866956815865 801.125878987934 813.153434705284;720.044246232086 720.044246232086 742.866930253765 747.250964575908 735.027333656649 719.577465323261 717.190065288522 731.346650709908 750.347138521549 763.475345837109 773.693695717131 789.287798577171 810.518185319644 830.111125982765 843.472450346469 853.378699854974;742.940029895664 742.940029895664 774.051061690388 778.109278632265 756.158768307305 729.133348286078 719.675868620086 730.858753459052 750.120917235613 769.107592698316 791.43919922736 819.937392622987 848.465639352439 869.583065525131 882.542471581944 891.497221184153;751.128194054408 751.128194054408 798.355948315463 811.118879495119 782.702971810268 740.991152302918 719.166629203507 720.779350853815 730.890274465969 743.244261352312 765.122077076672 800.206647211974 840.560759205098 875.885847376542 901.732073826025 918.7852989808;760.390444558366 760.390444558366 818.248253053742 845.893381243408 823.870331783674 775.723249240968 744.375936777649 739.212578761184 743.260884253152 746.991261909214 758.131435835839 784.685345060861 822.994274416249 863.420173507977 899.194387278248 928.155676508583;779.777710435288 779.777710435288 833.952124804665 868.444608317891 856.250939982233 810.055046298508 777.04925925875 770.612491616704 774.780790522025 779.677457818987 790.970686800993 812.992905723067 841.321530086259 871.578302755832 903.548891929093 936.612708265006;807.713277729328 807.713277729328 851.752038731432 878.642727733983 870.714120493806 837.921681313453 812.704397339618 807.096322838226 812.376612406267 822.880628995622 843.013341279409 870.747739453674 896.748815338628 919.669569756408 944.760710125872 972.156213958338;836.382966100616 836.382966100616 868.352453836189 887.487438000152 886.245819574568 869.191445492442 849.973347462264 842.20897598561 847.460859986976 863.343240359816 891.049687531691 925.768619729496 956.702124611688 980.35591352579 1001.44081730385 1022.73565285885;863.195224059471 863.195224059471 885.262751981801 898.5315406408 899.39976946196 889.472673987941 876.775165296379 872.27604543077 879.280482906539 896.737042025969 925.777063461042 962.385734081934 ...(+12237 chars)])  Name5=[300 300 300 300 300 300 300 300 300 300 300 300 300 300 300 300 300 300 300 300;297.183191911082 296.381813482439 298.389346568793 300 300 300 300 300 300 300 300 300 294.67266237158 289.737568904754 289.12856875624 291.461389167304 295.189395927038 297.348559050166 294.666946050542 286.881979097439;300 300 300 300 300 300 300 300 300 300 300 295.311694583484 288.854995920935 285.748220888279 286.130153267134 289.042144321121 293.243311010686 295.055826333218 287.545970834715 273.554783231216;300 300 300 300 298.49404534039 284.553749077953 261.448898184998 238.707345487409 254.949441131286 265.599575550091 295.677653030517 300 300 300 300 300 300 300 284.419815180476 261.388018187759;299.898205056662 292.176013706802 280.489559192747 273.801475207664 285.267789972213 268.982289185 248.031226594938 237.002933175585 247.269718357657 266.486860456224 296.010628081896 300 300 300 300 300 300 300 286.278851967763 251.317497463977;257.787117715529 230.011418991628 194.79567839807 217.609945177071 238.011497997128 244.713362579463 248.307562590703 254.695511354579 262.767152384925 269.435894142237 279.964353630393 300 300 300 300 300 300 300 300 252.247426167928;244.322164627464 226.527131172705 213.047581606847 208.860573467528 215.436572460517 230.257055418638 247.71372128472 261.030678888545 264.562685576978 255.804646726121 236.560489592442 212.844962970881 193.289036483877 186.243942541361 196.420463604227 222.426431060715 256.501420981836 286.894148423494 300 294.746256064465;219.827091553639 224.00842185519 226.545147573507 228.801538184105 231.197671510704 233.328041106659 234.425064195191 233.869076886551 231.523160498036 227.853678111254 223.908810740718 221.191949545254 221.375059646733 225.801644328901 234.876097447666 247.606442228722 261.586362170144 273.512050995951 280.050090404176 278.699668055487;253.235653200863 238.315624663681 223.001448394165 210.254255439123 202.14302656868 199.596251942444 202.290727140351 208.74083615883 216.703414841512 223.908681461858 228.900345602987 231.595168993526 233.230095692023 235.664906994489 240.366291593439 247.574154702973 256.032407983205 263.350862590025 266.765300968141 263.943316381967;248.250293366452 233.417397015265 222.629357327487 216.596802702064 214.504013108419 214.81806354172 216.051223315593 217.193946153414 217.807532354882 217.934808981726 217.977570533706 218.581966234929 220.499755224279 224.409471192001 230.735069374117 239.511489718516 250.303231623288 262.14379859624 273.489242792845 282.252586128849;242.086120224848 231.058285918819 223.245524598864 216.337716642453 212.00473270881 210.686778459967 211.585047714386 213.166686160244 214.004603934158 213.551990844805 212.439775437554 212.136104170727 214.180677075341 219.45152567214 227.861873339277 238.565025705036 250.403923777452 262.226566009688 272.865736774747 280.895220351927;240.36005533725 232.486162829539 226.900934366509 218.228275058477 210.073138425769 205.914056262523 206.863704975026 211.780406579307 218.363100263461 224.502124938947 229.114817814123 232.147403860389 234.026061788487 235.150186450836 235.841184590216 236.675239999685 238.744779946964 243.413612851756 251.528383016844 262.510332308677;239.698447912074 232.198026859744 223.919414459446 215.521411204134 208.833017267823 206.211824916001 207.251476971107 209.476538949511 210.219164042317 208.589475472156 206.308833127149 206.824526287407 213.201356834861 226.090216081071 243.04996560855 259.64415199246 271.618523010977 276.830575274702 275.838901872999 270.954993619848;239.699124464556 233.605232579107 228.311199393793 224.353241232463 217.305414394382 214.392354260996 217.338892875621 224.705113920913 232.919686598668 238.298745155624 238.931493145234 235.439120293715 230.335964150791 226.556951715392 226.115112416361 229.595190701737 236.519242380678 246.043219412989 257.344197449557 263.377380468519;239.816295103623 235.306294052789 231.603067258988 227.141295414711 219.929221129055 221.663517863192 223.173313363379 ...(+1903 chars)]  f_eff=f_eff  f_eff_3d=cat(3,[0 300 300 300 300 300 300 300 300 300 300 300 300 300 300 300;0 297.183191911082 296.426611034351 298.164901875909 299.729890418369 300 300 300 300 300 300 300 300 298.246280159588 293.323941175677 289.605177568121;0 300 300 300 300 300 300 300 300 300 300 300 298.194565616 293.186197508235 288.005939390271 285.831249666291;0 300 300 300 300 298.830780543781 288.45010517615 269.198351279529 247.606213934292 247.685895253279 260.241433389077 278.863820898602 297.342159316902 300 300 300;0 299.898205056662 292.607688999651 281.796119324753 274.923079354231 282.703893503121 273.534137231115 255.058291066139 241.31835233968 242.678361009153 256.818608841417 279.506658601707 297.54690795098 300 300 300;0 257.787117715529 231.564097802281 198.732841942692 213.783950127176 233.449660099476 242.840170615456 247.102054512399 252.195879229584 259.157474408621 266.080812885453 274.078879382355 287.67994415782 300 300 300;0 244.322164627464 227.521884595642 214.554611993092 209.56274253437 213.966162747799 226.114684405499 241.858690497339 255.819695478353 262.983154635567 260.210865029968 247.318092959095 227.427802322027 206.407297729817 191.363669195239 188.456229728941;0 219.827091553639 223.774682894234 226.261538486987 228.423137274253 230.66189014575 232.732596188535 234.057118563013 234.086637137758 232.572265963707 229.699815212679 226.114016103129 222.86256605675 221.252228025865 222.58480949776 227.774351528633;0 253.235653200863 239.149663526008 224.713592324918 212.391983450217 203.956717496232 200.308083359715 201.386990117451 206.216880455947 213.142510089008 220.283671547274 226.109974343971 229.938103678847 232.133374676882 233.89550996102 236.686947124696;0 248.250293366452 234.246565134276 223.835473565872 217.608473353533 214.971966061035 214.7302854703 215.63761693181 216.746793738614 217.53313355671 217.870775399277 217.953666560549 218.210319188835 219.213288076144 221.568249029122 225.784601231591;0 242.086120224848 231.674748706113 224.119001019729 217.496168908435 212.97359868155 211.055150765544 211.283764858867 212.547784159691 213.629882942097 213.779703020194 213.061510758378 212.322833707472 212.809162331873 215.621157437199 221.279862121518;0 240.36005533725 232.926318311337 227.525369846848 219.682696184669 211.896647238051 207.076532643554 206.545189257789 209.856479864588 215.41928693887 221.413547307181 226.536293846633 230.282645981008 232.7658440479 234.333275981924 235.300403437658;0 239.698447912074 232.617305055216 224.84497360979 216.929771998503 210.32855876911 206.944456318684 206.902773797345 208.605862523179 209.887058410752 209.409380901864 207.583726363488 206.507423039795 208.923731374457 216.723777995316 229.777118152262;0 239.699124464556 233.94588492053 228.90307888035 225.016998191195 218.881325985506 215.206563615048 216.350612843387 221.822679598842 229.246088879423 235.592510726348 238.57778308893 237.586604221047 233.759199327411 229.303190565961 226.460899693864;0 239.816295103623 235.558405912774 232.017092614817 227.889542866857 221.541858857525 221.178776539986 222.666922326049 223.807373577054 224.347949770768 224.2060554897 223.664268967536 223.317544283845 223.826730151672 225.633784301262 228.798384087427;0 239.0241787671 235.275750326049 231.884170916615 228.632534910313 225.682479941919 219.759890149376 214.807713434217 212.72031699795 213.270783872853 215.632967963887 218.814825174176 221.955375707671 224.402906794609 225.619645320011 225.039790135475;0 237.076762181258 233.090693425745 228.844528300962 223.574157582612 215.026904315874 203.385940748364 203.624488006545 208.887659548048 214.07458987715 219.17400417709 223.367403483949 225.215851514176 223.07095530856 218.631615953904 217.529914033361;0 234.418370415875 230.075356198925 225.110400190494 218.940110393671 211.545696211612 207.41906398842 212.230183010831 216.145170627157 216.881756265916 216.305112535715 214.160983315751 212.760331224129 212.920572248404 211.356342203357 211.033117448086;0 ...(+9495 chars)])  Name6=EO HC  f_hc=f_hc  f_hc_3d=cat(3,[0 5.41090940906478e-10 5.82277246149883e-10 6.06293368838046e-10 5.93131722841061e-10 5.23839609255542e-10 3.91944606807851e-10 2.09234652579032e-10 5.4438838779207e-11 0 0 0 0 0 0 8.76094213556711e-14;0 9.66157682132999e-10 1.14171380367877e-09 1.3085398373022e-09 1.436731750244e-09 1.50140710830807e-09 1.49054993471198e-09 1.4037387429616e-09 1.25592949365723e-09 1.08480750810599e-09 9.48415092070956e-10 9.01122102300235e-10 9.57886865196846e-10 1.07945131117581e-09 1.19756636123401e-09 1.25861853636732e-09;0 1.51893073819961e-09 1.87308690294655e-09 2.23556595270689e-09 2.57170270393273e-09 2.85154533221247e-09 3.04284043924759e-09 3.11378303127804e-09 3.05621981222313e-09 2.91369358374749e-09 2.78018397956802e-09 2.7564106348572e-09 2.87445960955754e-09 3.06205020857146e-09 3.1994920140049e-09 3.20815364803705e-09;0 2.18569631279908e-09 2.75719661582542e-09 3.3623976875487e-09 3.96646315092983e-09 4.52696347072398e-09 4.98270146550498e-09 5.26752335568588e-09 5.34710722375353e-09 5.26835363386512e-09 5.1685667326918e-09 5.20035067255693e-09 5.40754439909597e-09 5.67615476025969e-09 5.8306526872498e-09 5.77044430457704e-09;0 2.93480648169002e-09 3.73895205313518e-09 4.6062042207148e-09 5.50138385941712e-09 6.36410920761391e-09 7.11268314040406e-09 7.66396858697008e-09 7.95114359351344e-09 8.00028306393327e-09 7.99003135917068e-09 8.10873651384997e-09 8.39466551036389e-09 8.71884471834636e-09 8.87349612671262e-09 8.72142368435253e-09;0 3.7067767651549e-09 4.73712666955322e-09 5.86533360906322e-09 7.04304389488618e-09 8.18982467099753e-09 9.21394175771151e-09 1.00258735294025e-08 1.05431750459202e-08 1.07666342773999e-08 1.08579222871287e-08 1.10225829612807e-08 1.13476980417056e-08 1.17299839650705e-08 1.19079967161962e-08 1.16677397520458e-08;0 4.45361361921691e-09 5.70410931198504e-09 7.08297753126844e-09 8.52131372282291e-09 9.92420040629535e-09 1.11925722534742e-08 1.22279922485612e-08 1.29480699501458e-08 1.3336529992091e-08 1.34841507176011e-08 1.35673374840041e-08 1.37675961483196e-08 1.41174757467466e-08 1.43498742443037e-08 1.41124767213646e-08;0 5.16692255350104e-09 6.63486779588866e-09 8.25478576976627e-09 9.94152665401874e-09 1.15968258626344e-08 1.31207944055877e-08 1.44133720301719e-08 1.53829013457219e-08 1.59611687315809e-08 1.61214539178139e-08 1.59388703473217e-08 1.56748840607486e-08 1.56351428368566e-08 1.57984482916966e-08 1.58258294521693e-08;0 5.86534877365624e-09 7.55071115948705e-09 9.40787097124005e-09 1.13456659008478e-08 1.32706550483072e-08 1.50897433935242e-08 1.67089193800209e-08 1.80332771640949e-08 1.89598090090926e-08 1.93363133081943e-08 1.89983353938691e-08 1.81496744147917e-08 1.74956156045047e-08 1.7470024257118e-08 1.7696714242961e-08;0 6.57685280874934e-09 8.48097667547475e-09 1.05747569428809e-08 1.27675572172301e-08 1.49730139175668e-08 1.71084615905939e-08 1.90926302599686e-08 2.08422305614833e-08 2.22656507884058e-08 2.32058747104937e-08 2.32477944952659e-08 2.2304068979954e-08 2.11552729058493e-08 2.05998550325242e-08 2.05820544522234e-08;0 7.3259824175589e-09 9.44998964470792e-09 1.17778171467981e-08 1.42180585752055e-08 1.66864012910281e-08 1.91056950070265e-08 2.1403906536052e-08 2.3507547080697e-08 2.53203804938546e-08 2.66367435688037e-08 2.70678015448994e-08 2.64858874589515e-08 2.5424935203163e-08 2.4600876228137e-08 2.425936763944e-08;0 8.12528918056832e-09 1.04704886098662e-08 1.30276381594665e-08 1.56973012675808e-08 1.83858258459877e-08 2.10079836697361e-08 2.3485405703222e-08 2.57351525190534e-08 2.76409675552712e-08 2.90175271834415e-08 2.96610964565784e-08 2.95541757543508e-08 2.89914684566784e-08 2.83984507455331e-08 2.80528471875283e-08;0 8.96821536841883e-09 1.15374676635392e-08 1.43227594781306e-08 1.72079261525586e-08 2.00770427149229e-08 2.28225401631622e-08 2.53497819900165e-08 2.75714686803287e-08 2.93957617073589e-08 3.07271012722358e-08 3.15072489663473e-08 3.17836134024851e-08 3.17273192623881e-08 3.15604990385693e-08 3.14740678961609e-08;0 ...(+14592 chars)])  Name7=EO CO  f_co=f_co  f_co_3d=cat(3,[0 1.67160387663193e-08 1.20397081499173e-08 9.52610812306698e-09 8.36631447493353e-09 7.72547679934784e-09 6.8319182072918e-09 5.0682750909637e-09 2.053636244448e-09 2.64830540952401e-10 0 0 0 0 0 0;0 1.8291738663811e-08 1.5484401198941e-08 1.54411575714574e-08 1.72039510086271e-08 1.97426073770272e-08 2.2067112907845e-08 2.33532431661193e-08 2.30715889811663e-08 2.1102272015203e-08 1.7803239120534e-08 1.39825281296076e-08 1.07144428348684e-08 8.9547716217503e-09 8.97294518109532e-09 9.73626581616763e-09;0 1.89455854190192e-08 1.76213438227932e-08 1.98007712489662e-08 2.43781826914061e-08 3.01072238083766e-08 3.57321428517592e-08 4.01449190441459e-08 4.25615700206463e-08 4.27037393349085e-08 4.09540065447283e-08 3.84240381828016e-08 3.68405451230499e-08 3.81400263418887e-08 4.3714897490739e-08 5.34128678917819e-08;0 1.9707154323245e-08 1.92622231960563e-08 2.31867257121728e-08 3.02542190419942e-08 3.9015510929493e-08 4.79425656860809e-08 5.56069642044215e-08 6.08898431392073e-08 6.32177164272788e-08 6.28045112181993e-08 6.08454282535351e-08 5.95481786086419e-08 6.18231928510624e-08 7.0455124973334e-08 8.67424091607081e-08;0 2.23874366967191e-08 2.19430238033583e-08 2.67994727428016e-08 3.56655121600132e-08 4.69503954124918e-08 5.89158729012478e-08 6.98629035579479e-08 7.83506595202789e-08 8.34502814366758e-08 8.50330724818061e-08 8.40668098153838e-08 8.2821949470655e-08 8.47723422937577e-08 9.3886115536576e-08 1.13101927592328e-07;0 2.97014285217744e-08 2.80584900715061e-08 3.25872685992409e-08 4.20128136159412e-08 5.47129373499403e-08 6.88779250095538e-08 8.26960984262372e-08 9.45589808034902e-08 1.03289192284248e-07 1.08403144327939e-07 1.10416901193996e-07 1.11151455453234e-07 1.13858405154452e-07 1.22809143167723e-07 1.41954889939323e-07;0 4.52595059052667e-08 4.08955076377101e-08 4.33204620361185e-08 5.13741818461108e-08 6.35497911512864e-08 7.81597704000512e-08 9.35146955895325e-08 1.08106097195755e-07 1.20788125859134e-07 1.30956948536058e-07 1.38741367343936e-07 1.45219218790548e-07 1.52597918561019e-07 1.6410928892878e-07 1.83190076857492e-07;0 7.32895497038995e-08 6.44253688950243e-08 6.24791448563362e-08 6.65195513444765e-08 7.53282347674787e-08 8.75536782858015e-08 1.01864838444207e-07 1.17111810913705e-07 1.32484646506495e-07 1.47625834505435e-07 1.62646856206707e-07 1.78057139393369e-07 1.94684284919659e-07 2.13620186082007e-07 2.36012494248674e-07;0 1.17946941625535e-07 1.02691823332952e-07 9.37715168179527e-08 9.06264509776299e-08 9.25403757576405e-08 9.87278619345053e-08 1.0840144651812e-07 1.20882446632538e-07 1.35780906406612e-07 1.5315421386179e-07 1.73458188949641e-07 1.97164614072069e-07 2.24171933445419e-07 2.53396636984833e-07 2.82886445738555e-07;0 1.82210832581963e-07 1.58763539046906e-07 1.40207045169324e-07 1.26544117178008e-07 1.17854078776402e-07 1.14222322953281e-07 1.15593861801993e-07 1.2172825416754e-07 1.32393509968658e-07 1.47719084002419e-07 1.68364259121247e-07 1.95110088463916e-07 2.27847189329484e-07 2.64554761137194e-07 3.01192874704994e-07;0 2.66660905670144e-07 2.33521722877046e-07 2.02945929559443e-07 1.75730742252678e-07 1.53146902413632e-07 1.36611383557461e-07 1.27149890413182e-07 1.24990748892476e-07 1.29639930638478e-07 1.40484403360697e-07 1.57494255494365e-07 1.81316428520279e-07 2.1235937700989e-07 2.49336478987284e-07 2.88507413324858e-07;0 3.68689175545917e-07 3.24835446426624e-07 2.80458221695929e-07 2.37363481691102e-07 1.98449976650769e-07 1.67072510228093e-07 1.45949852412648e-07 1.36142919835525e-07 1.3674812110406e-07 1.45614327655155e-07 1.60715529989296e-07 1.8123602453498e-07 2.07487492943947e-07 2.39640853287404e-07 2.76348372004545e-07;0 4.82648398659756e-07 4.27652069852061e-07 3.68555055755657e-07 3.08270234930458e-07 2.5163385581579e-07 2.04494764547792e-07 1.72006398954068e-07 1.56803867431257e-07 1.58027822519984e-07 1.71848968403196e-07 1.93339806527179e-07 2.18693222283221e-07 2.4650223152165e-07 2.77420692697527e-07 3.12684816885102e-07;0 ...(+14605 chars)])  Name8=EO NOx  f_nox=f_nox  f_nox_3d=cat(3,[0 3.21218888850422e-07 1.79563354015778e-08 0 0 0 0 7.27128716806088e-09 2.382216838202e-07 4.44107113496821e-07 4.91577691057171e-07 5.14872133427744e-07 5.86973145400533e-07 7.14855423266785e-07 9.07945412418829e-07 1.1362893758644e-06;0 0 0 0 0 4.01712899078589e-07 9.14038671754761e-07 1.21206139039062e-06 1.258219700583e-06 1.15680571609299e-06 9.88518749662651e-07 7.9819948867334e-07 6.32587851093257e-07 5.69269922348739e-07 6.79185853795409e-07 9.13608733038228e-07;0 0 0 9.52027489513871e-08 8.30746833258196e-07 1.36030218646627e-06 1.73988427267659e-06 2.04152790117286e-06 2.20895266298404e-06 2.18125415927187e-06 1.94993025994388e-06 1.56653918990438e-06 1.12774239120503e-06 7.00461292902491e-07 3.43994753744295e-07 2.38110897923334e-07;0 0 1.31451622967041e-08 8.74752207158529e-07 1.77381400236465e-06 2.85505059786523e-06 3.97244136236958e-06 4.91927989175401e-06 5.50869973030963e-06 5.6102454452155e-06 5.18886396119566e-06 4.28820417240782e-06 3.03030934369309e-06 1.77477522325345e-06 9.94743171474735e-07 8.19166226001805e-07;0 0 8.46501289091852e-07 2.51723239043499e-06 4.63702986382199e-06 6.97443962050002e-06 9.24740955295268e-06 1.1057647942355e-05 1.20240484757528e-05 1.19560636442059e-05 1.07764628651257e-05 8.63325691824951e-06 6.10465785533055e-06 3.89116567479568e-06 2.39721925455604e-06 1.83191674225781e-06;0 8.04299318856711e-07 3.42277118336147e-06 6.71231990315139e-06 1.0496634563528e-05 1.42412740250893e-05 1.74585409927942e-05 1.98003313309143e-05 2.09159972358789e-05 2.03831613528198e-05 1.80395296628694e-05 1.43514937153895e-05 1.01802026481764e-05 6.39543568857852e-06 3.67625247299238e-06 2.17539035501076e-06;0 4.18403635223244e-06 8.53022483954423e-06 1.34771211881709e-05 1.85196642603013e-05 2.34006450258875e-05 2.77742815991628e-05 3.11840537431359e-05 3.30007063666191e-05 3.24628576710176e-05 2.91966375333571e-05 2.34144662842947e-05 1.62627968773842e-05 9.67259169011386e-06 5.07903152948792e-06 2.62351967770101e-06;0 9.6844239006658e-06 1.56670200795944e-05 2.17408858281583e-05 2.81317508143627e-05 3.46651103625967e-05 4.08469288470995e-05 4.60818070511369e-05 4.96401128612998e-05 5.06377854960177e-05 4.73209131871863e-05 3.83868097487482e-05 2.57581425208862e-05 1.43527195601674e-05 7.48773620062972e-06 4.12651812484211e-06;0 1.7217276591403e-05 2.38603432824287e-05 3.07464764538253e-05 3.87401399353274e-05 4.76303203786226e-05 5.64642244135301e-05 6.41543534687279e-05 7.09536645313842e-05 7.65440790256632e-05 7.62436421958216e-05 6.39802917080371e-05 4.07630432911696e-05 2.01835393277083e-05 1.27322489675938e-05 8.34894165677621e-06;0 2.59973378464546e-05 3.17138915815894e-05 3.89110422231306e-05 4.90429961790851e-05 6.16533321661544e-05 7.47993558030312e-05 8.64012220043849e-05 9.73063735753573e-05 0.000110954137979213 0.000119740220882612 0.000108840097128983 7.66374544495414e-05 4.23916089474961e-05 2.38571863874159e-05 1.56502938279821e-05;0 2.94701264228928e-05 3.6213230815927e-05 4.41277150128939e-05 5.73373909243478e-05 7.61007798922144e-05 9.57613713660942e-05 0.000113612141664159 0.00013096766174073 0.000149883585738345 0.0001644325988204 0.000152261866724626 0.000103999486884709 5.31185248454306e-05 3.21668594322779e-05 2.38194668762723e-05;0 3.35185356614725e-05 4.11284242733725e-05 4.78301786308674e-05 6.28516991863075e-05 9.27665504900369e-05 0.000119587353496318 0.000139413430726879 0.000154148371733834 0.000163513627860459 0.000163616314711516 0.000141940939447349 9.54283151265787e-05 5.37322316241257e-05 4.11532599321637e-05 3.35586455204069e-05;0 4.18588832755133e-05 5.30156550779618e-05 6.5453764267152e-05 8.76863772443697e-05 0.000124525228002101 0.00014865354394301 0.000163772828471961 0.000172185888447209 0.000169441116848506 0.00014928131460553 0.000120407776087826 9.7839420186128e-05 7.94472650211143e-05 5.86533438484391e-05 4.44488942287757e-05;0 5.26473524639921e-05 6.8752348897689e-05 8.82510579878347e-05 0.000113462966789653 0.000142289957668836 ...(+14258 chars)])  Name9=EO CO2  f_co2=f_co2  f_co2_3d=cat(3,[0 0 0 0 0 0 0 0 0 0 0 0 0 0 0 0;0 0 0.00030365633115907 0.000477004645283182 0.000566806090053379 0.000616848625254133 0.000657878888237009 0.000704613499127597 0.000759308138241543 0.000818372753847269 0.000877510431637555 0.00093411034677875 0.000987559137783125 0.00103750226880644 0.00108100059676674 0.00111208043085771;0 0.000531197372565358 0.000833769373636657 0.00101208952923391 0.00111931128184282 0.00120336184488415 0.00129722537528743 0.00140997808510818 0.00153485003497759 0.00166189835257539 0.00178421226628486 0.00189870859123887 0.00200545899125166 0.00210557816401844 0.00219673582357201 0.00227206518127521;0 0.000875228699122675 0.00120046009101224 0.00142093976501899 0.00158063459786091 0.00172698904223179 0.00189805820656259 0.0020934657211037 0.0022961483011719 0.00249286148581882 0.00267768820840761 0.00284908873634617 0.00300734462013376 0.00315199589511178 0.00327966962842089 0.00338565128082482;0 0.00112894236857282 0.00150365338268639 0.00179791598213576 0.00204513432594278 0.00228381248652535 0.00254264495809689 0.0028157705345395 0.00308495797525869 0.00333949093420176 0.00357682369134973 0.00379724326119826 0.0040004288745128 0.00418332550924124 0.00434015076880871 0.00446687499014148;0 0.0013694514734865 0.00181255663935764 0.00219736379952817 0.00254899113243675 0.00289243842715691 0.00323933383331892 0.00357940420638906 0.00389996239244074 0.00419834718509891 0.00447662773375111 0.0047360527393408 0.00497566516999516 0.00519105062075714 0.00537417147233103 0.00551962844763135;0 0.00163396590821415 0.0021504690371032 0.00262305920229874 0.00307027998441048 0.00350564168807108 0.00393090022171935 0.00433360227070106 0.00470487512701578 0.00504653382575368 0.00536303791746496 0.00565641037717889 0.00592599316976571 0.00616798777596206 0.00637647593791359 0.00654882383360534;0 0.00191645826900269 0.00250624896727007 0.00305843491314744 0.0035867469936911 0.0040978426589801 0.00458941140866771 0.00505272199035049 0.00548106070220549 0.0058737454392985 0.00623337644778486 0.00656257310986629 0.00686262794236557 0.00713298321204598 0.00737195752566903 0.00757987146027694;0 0.00220779503528263 0.00286778580188851 0.00349257477090796 0.00409286732910444 0.00467250391062088 0.0052286435941315 0.00575451835386064 0.00624375391440032 0.00669300479035286 0.00710199609710946 0.00747273402813795 0.00780885364227351 0.00811413326375108 0.00839067570230487 0.00863997981618954;0 0.00250378076698133 0.00323101071266567 0.00392425352797351 0.00459300986818308 0.00524037037011277 0.00586351401735864 0.00645604739002077 0.00701097061645394 0.00752279816639411 0.00798854348211049 0.00840846220761616 0.00878733069903513 0.00913311248052539 0.00945114923691524 0.00974240584364766;0 0.00280475043657424 0.00359767354395676 0.00435752073541733 0.00509407292037811 0.00581057029372124 0.00650380309382036 0.00716680271655133 0.00779176543139013 0.00837192879417746 0.00890250193469743 0.00938152566113212 0.00981171888076588 0.0102004875265908 0.0105552451871903 0.0108809264574539;0 0.00311346404921585 0.00397249731054076 0.00479865853976343 0.00560316562677121 0.00638996643253621 0.00715444869369664 0.00788836214979145 0.0085832505109625 0.00923207032274121 0.00982966447392534 0.0103723919601302 0.0108580664514062 0.0112881736128468 0.0116712180554654 0.0120221656588126;0 0.00343191752302102 0.00436015298219231 0.00525476525032292 0.00612780499681866 0.00698388792273074 0.00781670284852585 0.00861665792448635 0.00937424346968913 0.0100819170973999 0.010735101618821 0.0113308925287724 0.0118640528063634 0.0123297417735677 0.01273739279869 0.0131136804400777;0 0.00375693708520568 0.00475886927039337 0.00572609606973659 0.00666900284845912 0.00759094499421124 0.00848662498834914 0.0093454304072657 0.0101549494758421 0.0109044992901486 0.0115885489732343 0.0122076018867566 0.012763057986659 0.0132552948646921 0.013696267711973 0.0141140170711275;0 0.00407804884129998 0.00515634246179069 0.00619725237396766 0.00720963330551028 ...(+12973 chars)])  Name10=Brake Torque  f_pm=f_pm  f_pm_3d=cat(3,[0 0 0 0 0 0 0 0 0 0 0 0 0 0 0 0;0 0 0 0 0 0 0 0 0 0 0 0 0 0 0 0;0 0 0 0 0 0 0 0 0 0 0 0 0 0 0 0;0 0 0 0 0 0 0 0 0 0 0 0 0 0 0 0;0 0 0 0 0 0 0 0 0 0 0 0 0 0 0 0;0 0 0 0 0 0 0 0 0 0 0 0 0 0 0 0;0 0 0 0 0 0 0 0 0 0 0 0 0 0 0 0;0 0 0 0 0 0 0 0 0 0 0 0 0 0 0 0;0 0 0 0 0 0 0 0 0 0 0 0 0 0 0 0;0 0 0 0 0 0 0 0 0 0 0 0 0 0 0 0;0 0 0 0 0 0 0 0 0 0 0 0 0 0 0 0;0 0 0 0 0 0 0 0 0 0 0 0 0 0 0 0;0 0 0 0 0 0 0 0 0 0 0 0 0 0 0 0;0 0 0 0 0 0 0 0 0 0 0 0 0 0 0 0;0 0 0 0 0 0 0 0 0 0 0 0 0 0 0 0;0 0 0 0 0 0 0 0 0 0 0 0 0 0 0 0;0 0 0 0 0 0 0 0 0 0 0 0 0 0 0 0;0 0 0 0 0 0 0 0 0 0 0 0 0 0 0 0;0 0 0 0 0 0 0 0 0 0 0 0 0 0 0 0;0 0 0 0 0 0 0 0 0 0 0 0 0 0 0 0],[0 0 0 0 0 0 0 0 0 0 0 0 0 0 0 0;0 0 0 0 0 0 0 0 0 0 0 0 0 0 0 0;0 0 0 0 0 0 0 0 0 0 0 0 0 0 0 0;0 0 0 0 0 0 0 0 0 0 0 0 0 0 0 0;0 0 0 0 0 0 0 0 0 0 0 0 0 0 0 0;0 0 0 0 0 0 0 0 0 0 0 0 0 0 0 0;0 0 0 0 0 0 0 0 0 0 0 0 0 0 0 0;0 0 0 0 0 0 0 0 0 0 0 0 0 0 0 0;0 0 0 0 0 0 0 0 0 0 0 0 0 0 0 0;0 0 0 0 0 0 0 0 0 0 0 0 0 0 0 0;0 0 0 0 0 0 0 0 0 0 0 0 0 0 0 0;0 0 0 0 0 0 0 0 0 0 0 0 0 0 0 0;0 0 0 0 0 0 0 0 0 0 0 0 0 0 0 0;0 0 0 0 0 0 0 0 0 0 0 0 0 0 0 0;0 0 0 0 0 0 0 0 0 0 0 0 0 0 0 0;0 0 0 0 0 0 0 0 0 0 0 0 0 0 0 0;0 0 0 0 0 0 0 0 0 0 0 0 0 0 0 0;0 0 0 0 0 0 0 0 0 0 0 0 0 0 0 0;0 0 0 0 0 0 0 0 0 0 0 0 0 0 0 0;0 0 0 0 0 0 0 0 0 0 0 0 0 0 0 0],[0 0 0 0 0 0 0 0 0 0 0 0 0 0 0 0;0 0 0 0 0 0 0 0 0 0 0 0 0 0 0 0;0 0 0 0 0 0 0 0 0 0 0 0 0 0 0 0;0 0 0 0 0 0 0 0 0 0 0 0 0 0 0 0;0 0 0 0 0 0 0 0 0 0 0 0 0 0 0 0;0 0 0 0 0 0 0 0 0 0 0 0 0 0 0 0;0 0 0 0 0 0 0 0 0 0 0 0 0 0 0 0;0 0 0 0 0 0 0 0 0 0 0 0 0 0 0 0;0 0 0 0 0 0 0 0 0 0 0 0 0 0 0 0;0 0 0 0 0 0 0 0 0 0 0 0 0 0 0 0;0 0 0 0 0 0 0 0 0 0 0 0 0 0 0 0;0 0 0 0 0 0 0 0 0 0 0 0 0 0 0 0;0 0 0 0 0 0 0 0 0 0 0 0 0 0 0 0;0 0 0 0 0 0 0 0 0 0 0 0 0 0 0 0;0 0 0 0 0 0 0 0 0 0 0 0 0 0 0 0;0 0 0 0 0 0 0 0 0 0 0 0 0 0 0 0;0 0 0 0 0 0 0 0 0 0 0 0 0 0 0 0;0 0 0 0 0 0 0 0 0 0 0 0 0 0 0 0;0 0 0 0 0 0 0 0 0 0 0 0 0 0 0 0;0 0 0 0 0 0 0 0 0 0 0 0 0 0 0 0])  aMode=1  CalMapsFuelCmdData={'', '', 'MappedEngine-Torque', 'MappedEngine-Nonfiring'}  CalMapsTrqCmdData={'', '', 'MappedEngine-Torque', 'MappedEngine-Nonfiring'}
      settings: SourceProductBaseCode=PW,DR,MT,UV,VE
  Mux{,1..3} (4 alike) : Mux  Inputs=1
  Product : Product
  Terminator{,1,4..5,10,12..13} (7 alike) : Terminator
  EngTrq : Outport  Unit=N*m  VectorParamsAs1DForOutWhenUnconnected=off
  EngSpdOut : Outport  Port=2  VectorParamsAs1DForOutWhenUnconnected=off
  Map : Outport  Port=3  Unit=Pa  VectorParamsAs1DForOutWhenUnconnected=off
  Mat : Outport  Port=4  Unit=K  VectorParamsAs1DForOutWhenUnconnected=off
  ThrPosPct : Outport  Port=5  VectorParamsAs1DForOutWhenUnconnected=off
  WgAreaPct : Outport  Port=6  VectorParamsAs1DForOutWhenUnconnected=off
  IntkCamPhase : Outport  Port=7  VectorParamsAs1DForOutWhenUnconnected=off
  ExhCamPhase : Outport  Port=8  VectorParamsAs1DForOutWhenUnconnected=off
  TurboRackPos : Outport  Port=9  VectorParamsAs1DForOutWhenUnconnected=off
  EgrVlvAreaPct : Outport  Port=10  VectorParamsAs1DForOutWhenUnconnected=off
  VarCompRatioPos : Outport  Port=11  VectorParamsAs1DForOutWhenUnconnected=off
  IntkVlvLift : Outport  Port=12  VectorParamsAs1DForOutWhenUnconnected=off
  VarIntkRunLen : Outport  Port=13  VectorParamsAs1DForOutWhenUnconnected=off
  IntkSwirlVlvPos : Outport  Port=14  VectorParamsAs1DForOutWhenUnconnected=off
  FuelFlw : Outport  Port=15  VectorParamsAs1DForOutWhenUnconnected=off
  FuelVolFlw : Outport  Port=16  VectorParamsAs1DForOutWhenUnconnected=off
  IntkPortFlw : Outport  Port=17  VectorParamsAs1DForOutWhenUnconnected=off
  NormAirChrg : Outport  Port=18  VectorParamsAs1DForOutWhenUnconnected=off
  ExhManGasTemp : Outport  Port=19  VectorParamsAs1DForOutWhenUnconnected=off
  Afr : Outport  Port=20  Unit=1  VectorParamsAs1DForOutWhenUnconnected=off
  TurboSpd : Outport  Port=21  Unit=rad/s  VectorParamsAs1DForOutWhenUnconnected=off
  TurbPrsRatio : Outport  Port=22  Unit=1  VectorParamsAs1DForOutWhenUnconnected=off
  CompPrsRatio : Outport  Port=23  Unit=1  VectorParamsAs1DForOutWhenUnconnected=off
  TurbTempOut : Outport  Port=24  Unit=K  VectorParamsAs1DForOutWhenUnconnected=off
  CompTempOut : Outport  Port=25  Unit=K  VectorParamsAs1DForOutWhenUnconnected=off
  EgrPct : Outport  Port=26  Unit=%  VectorParamsAs1DForOutWhenUnconnected=off
  EgrMassFlwRate : Outport  Port=27  Unit=kg/s  VectorParamsAs1DForOutWhenUnconnected=off
  EgrCoolerTempOut : Outport  Port=28  Unit=K  VectorParamsAs1DForOutWhenUnconnected=off
  IntercoolerTempOut : Outport  Port=29  Unit=K  VectorParamsAs1DForOutWhenUnconnected=off
  BSFC : Outport  Port=30  VectorParamsAs1DForOutWhenUnconnected=off
  TP HC : Outport  Port=31  VectorParamsAs1DForOutWhenUnconnected=off
  TP CO : Outport  Port=32  VectorParamsAs1DForOutWhenUnconnected=off
  TP NOx : Outport  Port=33  VectorParamsAs1DForOutWhenUnconnected=off
  TP CO2 : Outport  Port=34  VectorParamsAs1DForOutWhenUnconnected=off
  Iat : Outport  Port=35  Unit=K  VectorParamsAs1DForOutWhenUnconnected=off
  Ect : Outport  Port=36  Unit=K  VectorParamsAs1DForOutWhenUnconnected=off
  EgrVlvDeltaPrs : Outport  Port=37  Unit=Pa  VectorParamsAs1DForOutWhenUnconnected=off
  EgrVlvInTemp : Outport  Port=38  Unit=K  VectorParamsAs1DForOutWhenUnconnected=off
  CylPrs : Outport  Port=39  VectorParamsAs1DForOutWhenUnconnected=off
  EngTrqCrk : Outport  Port=40  VectorParamsAs1DForOutWhenUnconnected=off
  CrkAng : Outport  Port=41  VectorParamsAs1DForOutWhenUnconnected=off
  wires:
  InjPw/1 -> Actuators/3(InjPwCmd)
  EngSpd/1 -> Accessory Load Model/2(EngSpd), Mapped CI Engine/2
  Accessory Load Model/2(EngTrqOut) -> EngTrq/1  "EngTrq"
  Product/1 -> Mapped CI Engine/1
  Injector Slope/1 -> Product/2
  AmbTemp/1 -> Terminator12/1
  Mapped CI Engine/1 -> Bus Selector/1
  Ground/1 -> Map/1
  Ground1/1 -> Mat/1
  TrqCmd/1 -> Terminator10/1
  AmbPrs/1 -> Terminator13/1
  UndHdFlwVel/1 -> Terminator4/1
  Bus Selector/6 -> ExhManGasTemp/1  "<ExhManGasTemp>"
  Bus Selector/7 -> Afr/1  "<Afr>"
  Bus Selector/1 -> EngSpdOut/1  "<EngSpd>"
  Bus Selector/2 -> FuelFlw/1  "<FuelMassFlw>"
  Bus Selector/4 -> IntkPortFlw/1  "<IntkGasMassFlw>"
  Bus Selector/9 -> Mux3/1  "<EoHC>"
  Bus Selector/10 -> Mux/1  "<EoCO>"
  Bus Selector/11 -> Mux1/1  "<EoNOx>"
  Bus Selector/12 -> Mux2/1  "<EoCO2>"
  Mux3/1 -> TP HC/1
  Mux/1 -> TP CO/1
  Mux1/1 -> TP NOx/1
  Mux2/1 -> TP CO2/1
  Bus Selector/8 -> BSFC/1  "<Bsfc>"
  Bus Selector/5 -> NormAirChrg/1  "<NrmlzdAirChrg>"
  Ground8/1 -> TurboSpd/1
  Ground9/1 -> TurbPrsRatio/1
  Ground10/1 -> CompPrsRatio/1
  Ground11/1 -> TurbTempOut/1
  Ground12/1 -> CompTempOut/1
  Ground13/1 -> IntercoolerTempOut/1
  Ground14/1 -> EgrPct/1
  Ground15/1 -> EgrMassFlwRate/1
  Ground16/1 -> EgrCoolerTempOut/1
  Injector Pulsewidth Dynamics/1 -> Product/1
  ThrPosPctCmd/1 -> Actuators/1(ThrPosPctCmd)
  WgAreaPctCmd/1 -> Actuators/2(WgAreaPctCmd)
  Actuators/3(InjPw) -> Injector Pulsewidth Dynamics/1
  Actuators/1(ThrPosPct) -> ThrPosPct/1
  Actuators/2(WgAreaPct) -> WgAreaPct/1
  Actuators/4(FuelMainSoi) -> Terminator5/1
  FuelMainSoi/1 -> Actuators/4(FuelMainSoiCmd)
  SpkAdv/1 -> Actuators/5(SpkAdvCmd)
  IntkCamPhaseCmd/1 -> Actuators/6(IntkCamPhaseCmd)
  ExhCamPhaseCmd/1 -> Actuators/7(ExhCamPhaseCmd)
  TurboRackPosCmd/1 -> Actuators/8(TurboRackPosCmd)
  EgrVlvAreaPctCmd/1 -> Actuators/9(EgrVlvAreaPctCmd)
  VarCompRatioPosCmd/1 -> Actuators/10(VarCompRatioPosCmd)
  IntkVlvLiftCmd/1 -> Actuators/11(IntkVlvLiftCmd)
  VarIntkRunLenCmd/1 -> Actuators/12(VarIntkRunLenCmd)
  ClsdLpFuelMult/1 -> Terminator1/1
  IntkSwirlVlvPosCmd/1 -> Actuators/13(IntkSwirlVlvPosCmd)
  Actuators/12(IntkSwirlVlvPos) -> IntkSwirlVlvPos/1
  Actuators/10(IntkVlvLift) -> IntkVlvLift/1
  Actuators/9(VarCompRatioPos) -> VarCompRatioPos/1
  Actuators/8(EgrVlvAreaPct) -> EgrVlvAreaPct/1
  Actuators/7(TurboRackPos) -> TurboRackPos/1
  Actuators/6(ExhCamPhase) -> ExhCamPhase/1
  Actuators/5(IntkCamPhase) -> IntkCamPhase/1
  Actuators/11(VarIntkRunLen) -> VarIntkRunLen/1
  Constant/1 -> Ect/1
  Ground3/1 -> EgrVlvDeltaPrs/1
  Ground2/1 -> EgrVlvInTemp/1
  Ground4/1 -> Iat/1
  Mapped CI Engine/2 -> Accessory Load Model/1(EngTrqIn)
  Accessory Load Model/1(PwrInfo) -> Terminator/1
  Bus Selector/3 -> FuelVolFlw/1  "<FuelVolFlw>"
  Ground5/1 -> CylPrs/1
  Ground6/1 -> EngTrqCrk/1
  Ground7/1 -> CrkAng/1
